simulink model "WL_test"  (R2025a)
settings: Solver=ode4  StartTime=0.0  StopTime=T_sim  FixedStep=Dt_sim  RelTol=1e-3
InitFcn:
  | % --- AVVIO AUTOMATICO PYTHON SERVER CON POP-UP (METODO FILE ROBUSTO) ---
  | fprintf('[Simulink] Preparazione simulazione...\n');
  | 
  | % 1. Pop-up per la Raffica
  | scelta_gust = questdlg('Vuoi includere la raffica (gust_H40.gust)?', ...
  |     'Configurazione Raffica', 'Si', 'No', 'No');
  | if isempty(scelta_gust), scelta_gust = 'No'; end
  | 
  | % 2. Pop-up per il Video
  | scelta_video = questdlg('Vuoi generare il video MP4 a fine simulazione?', ...
  |     'Configurazione Video', 'Si', 'No', 'No');
  | if isempty(scelta_video), scelta_video = 'No'; end
  | 
  | % --- PERCORSO ASSOLUTO ---
  | % Definiamo subito la cartella così MATLAB e WSL salvano e leggono dallo stesso posto
  | percorso = '/home/lpmatteo/Internship_INCARBONE_2026/LQR_first_controller_study/LQR_WL_simulation';
  | file_inputs = fullfile(percorso, 'python_inputs.txt');
  | 
  | % --- CREAZIONE FILE DI INPUT ---
  | fid = fopen(file_inputs, 'w');
  | fprintf(fid, '1\n'); % Scelta controller: 1 (LQI)
  | 
  | if strcmp(scelta_gust, 'Si')
  |     fprintf(fid, 's\n');
  | else
  |     fprintf(fid, 'n\n');
  | end
  | 
  | if strcmp(scelta_video, 'Si')
  |     % Se vogliamo il video, precompiliamo anche formato (mp4), qualità (high)
  |     % e la "Y" finale per far partire il render ASWING in automatico.
  |     fprintf(fid, 's\ngif\nmedium\nY\n');
  | else
  |     fprintf(fid, 'n\n');
  | end
  | fclose(fid);
  | 
  | % --- AVVIO DEL SERVER WSL ---
  | % Diciamo a Python di prendere le risposte direttamente dal file appena creato
  | cmd_wsl = sprintf('start "WingLoop Python Server" wsl -e bash -ic "cd %s && conda activate WINGLOOP && python3 controller_wingloop.py < python_inputs.txt; exec bash"', percorso);
  | 
  | system(cmd_wsl);
values from neighbouring files (symbols this model uses):
  E2ref = 23.6475887    [WL_main.m]
  F2ref = -6.63806152    [WL_main.m]
  t_int = 0.5    [WL_main.m]
  tau = 0.1    [WL_main.m]
  u_trim = [0, F2ref, F3ref, 0, E2ref, E2ref]    [WL_main.m]
undefined symbols (not defined in the file or in its folder): DiscIntNeverNeededParam, FullModel, idx, K_i, K_wu, K_z, matrices, ref_vec, ref_vecP, ROM, sat_engine
libraries: cstblocks x1
settings Model: SimulationMode=accelerator  Creator=lpmat  LastModifiedBy=lpmat

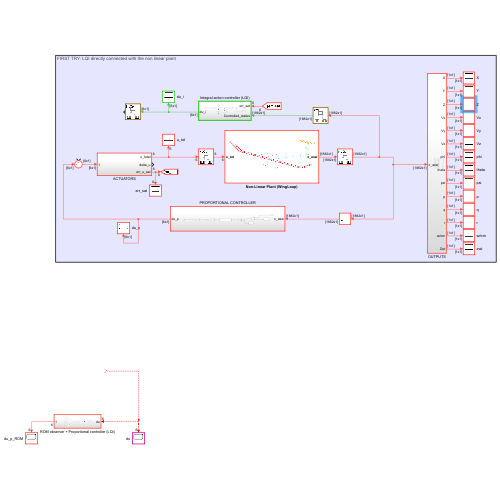
[thumbnail: Simulink's stored preview of the top-level diagram]
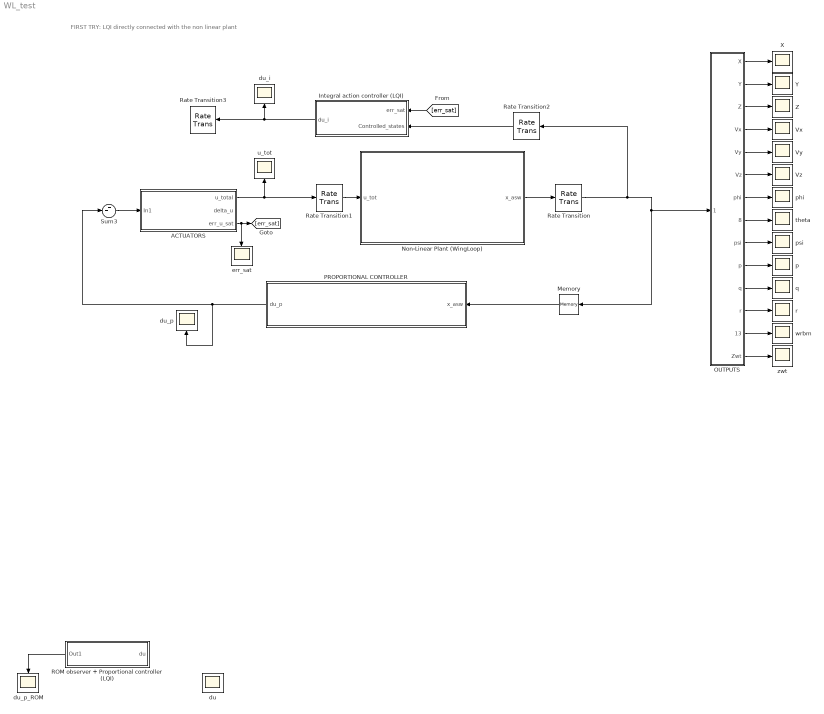
== system WL_test ==
  note: FIRST TRY: LQI directly connected with the non linear plant
  ACTUATORS : Subsystem
  Integral action controller (LQI) : Subsystem  TreatAsAtomicUnit=on  SystemSampleTime=t_int
  Memory : Memory  InitialCondition=FullModel.X0
  Non-Linear Plant (WingLoop) : Subsystem
      mask Display: image('Screenshot 2026-03-18 123158.png');
  OUTPUTS : Subsystem
  PROPORTIONAL CONTROLLER : Subsystem
  ROM observer + Proportional controller (LQI) : Subsystem
  Rate Transition : RateTransition  InitialCondition=FullModel.X0  OutPortSampleTime=Ts_control
  Rate Transition1 : RateTransition  InitialCondition=u_trim  OutPortSampleTime=Dt_asw
  Rate Transition2 : RateTransition  InitialCondition=FullModel.X0  OutPortSampleTime=t_int
  Rate Transition3 : RateTransition  OutPortSampleTime=Ts_control
  Sum3 : Sum  Inputs=--|
  Vx : Scope
      settings: ActiveDisplayYMinimum=-30.667463075  ActiveDisplayYMaximum=-29.643238325000002  DataLoggingVariableName=ScopeData9
  Vy : Scope
      settings: ActiveDisplayYMinimum=-0.022981843775  ActiveDisplayYMaximum=0.019016099975  DataLoggingVariableName=ScopeData2
  Vz : Scope
      settings: ActiveDisplayYMinimum=-4.1942458462499994  ActiveDisplayYMaximum=3.14147451625  DataLoggingVariableName=ScopeData23
  X : Scope
      settings: ActiveDisplayYMinimum=-3445.898072785  ActiveDisplayYMaximum=379.55975506499993
  Y : Scope
      settings: ActiveDisplayYMinimum=-11.715700294646378  ActiveDisplayYMaximum=7.8645535005168945
  Z : Scope
      settings: ActiveDisplayYMinimum=-2.916242765  ActiveDisplayYMaximum=10.900665085  DataLoggingVariableName=ScopeData11
  du : Scope
      settings: ActiveDisplayYMinimum=-1  ActiveDisplayYMaximum=1  DataLoggingVariableName=ScopeData15
  du_i : Scope
      settings: ActiveDisplayYMinimum=-0.0019582531234373637  ActiveDisplayYMaximum=0.0017838770388506043  DataLoggingVariableName=ScopeData5
  du_p : Scope
      settings: ActiveDisplayYMinimum=-2.2212573201433456  ActiveDisplayYMaximum=2.0941100207489196  DataLoggingVariableName=ScopeData13
  du_p_ROM : Scope
      settings: ActiveDisplayYMinimum=-1  ActiveDisplayYMaximum=1  DataLoggingVariableName=ScopeData10
  err_sat : Scope
      settings: ActiveDisplayYMinimum=-1  ActiveDisplayYMaximum=1  DataLoggingVariableName=ScopeData6
  p : Scope
      settings: ActiveDisplayYMinimum=-0.0001631406245  ActiveDisplayYMaximum=0.0001678073805  DataLoggingVariableName=ScopeData7
  phi : Scope
      settings: ActiveDisplayYMinimum=-4.954931666598749E-6  ActiveDisplayYMaximum=4.4625239296288751E-5  DataLoggingVariableName=ScopeData3
  psi : Scope
      settings: ActiveDisplayYMinimum=-2.941824858275E-5  ActiveDisplayYMaximum=3.8845402447499991E-6  DataLoggingVariableName=ScopeData4
  q : Scope
      settings: ActiveDisplayYMinimum=-0.1020126258875  ActiveDisplayYMaximum=0.12159143298749998  DataLoggingVariableName=ScopeData25
  r : Scope
      settings: ActiveDisplayYMinimum=-9.1499201112499989E-7  ActiveDisplayYMaximum=3.502066890125E-6  DataLoggingVariableName=ScopeData8
  theta : Scope
      settings: ActiveDisplayYMinimum=-0.557096708875  ActiveDisplayYMaximum=0.62679834987499994  DataLoggingVariableName=ScopeData14
  u_tot : Scope
      settings: ActiveDisplayYMinimum=-15.360293933915493  ActiveDisplayYMaximum=27.981801998175822  DataLoggingVariableName=ScopeData12
  wrbm : Scope
      settings: ActiveDisplayYMinimum=4.1562448775  ActiveDisplayYMaximum=36.6690849025  DataLoggingVariableName=ScopeData26
  zwt : Scope
      settings: ActiveDisplayYMinimum=2.5963466775  ActiveDisplayYMaximum=6.8764531025  DataLoggingVariableName=ScopeData16
  wires:
  Integral action controller (LQI)/1(du_i) -> Rate Transition3/1, du_i/1
  OUTPUTS/3(Z) -> Z/1
  OUTPUTS/4(Vx) -> Vx/1
  ACTUATORS/1(u_total) -> Rate Transition1/1, u_tot/1
  [err_sat] -> Integral action controller (LQI)/1(err_sat)
  Non-Linear Plant (WingLoop)/1(x_asw) -> Rate Transition/1
  OUTPUTS/8(theta) -> theta/1
  OUTPUTS/6(Vz) -> Vz/1
  OUTPUTS/11(q) -> q/1
  OUTPUTS/13(wrbm) -> wrbm/1
  OUTPUTS/1(X) -> X/1
  OUTPUTS/2(Y) -> Y/1
  OUTPUTS/5(Vy) -> Vy/1
  OUTPUTS/7(phi) -> phi/1
  OUTPUTS/9(psi) -> psi/1
  OUTPUTS/10(p) -> p/1
  OUTPUTS/12(r) -> r/1
  ACTUATORS/3(err_u_sat) -> err_sat/1, [err_sat]
  Rate Transition/1 -> Memory/1, OUTPUTS/1(x_asw), Rate Transition2/1
  Rate Transition1/1 -> Non-Linear Plant (WingLoop)/1(u_tot)
  ROM observer + Proportional controller (LQI)/1(Out1) -> du_p_ROM/1
  ? -> ROM observer + Proportional controller (LQI)/1(du), du/1
  PROPORTIONAL CONTROLLER/1(du_p) -> Sum3/2, du_p/1
  OUTPUTS/14(Zwt) -> zwt/1
  Rate Transition2/1 -> Integral action controller (LQI)/2(Controlled_states)
  Memory/1 -> PROPORTIONAL CONTROLLER/1(x_asw)
  Sum3/1 -> ACTUATORS/1(In1)

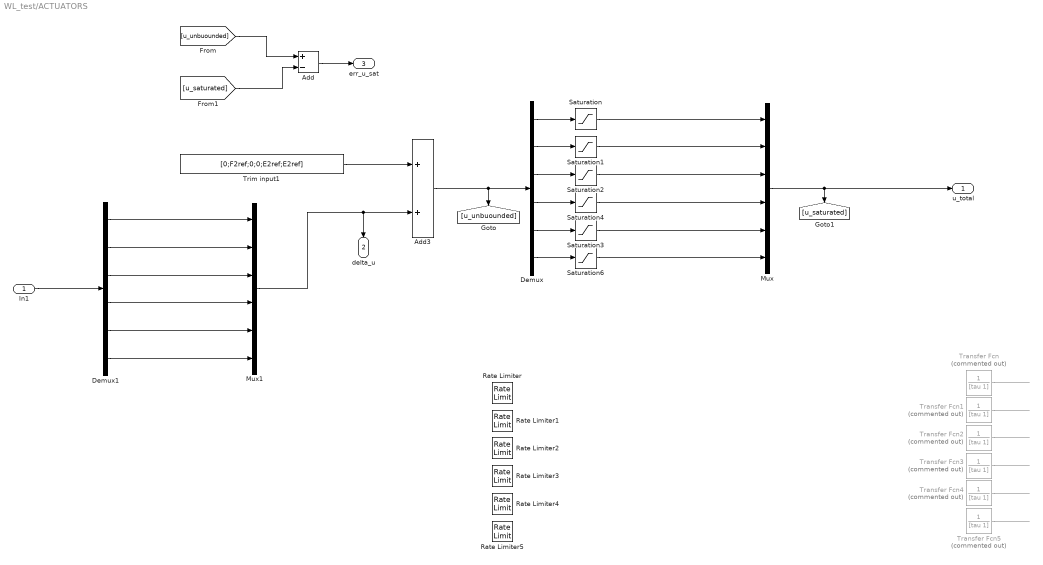
== system WL_test/ACTUATORS ==
  In1 : Inport
  Add : Sum  Inputs=+-
  Add3 : Sum
  Demux : Demux  Outputs=6
  Demux1 : Demux  Outputs=6
  Mux : Mux  Inputs=6
  Mux1 : Mux  Inputs=6
  Rate Limiter : RateLimiter  RisingSlewLimit=15  FallingSlewLimit=-15  SampleTimeMode=inherited  InitialCondition=u_trim(1)
  Rate Limiter1 : RateLimiter  RisingSlewLimit=15  FallingSlewLimit=-15  SampleTimeMode=inherited  InitialCondition=u_trim(2)
  Rate Limiter2 : RateLimiter  RisingSlewLimit=15  FallingSlewLimit=-15  SampleTimeMode=inherited  InitialCondition=u_trim(3)
  Rate Limiter3 : RateLimiter  RisingSlewLimit=15  FallingSlewLimit=-15  SampleTimeMode=inherited  InitialCondition=u_trim(4)
  Rate Limiter4 : RateLimiter  RisingSlewLimit=15  FallingSlewLimit=-15  SampleTimeMode=inherited  InitialCondition=u_trim(5)
  Rate Limiter5 : RateLimiter  RisingSlewLimit=15  FallingSlewLimit=-15  SampleTimeMode=inherited  InitialCondition=u_trim(6)
  Saturation{,1..2,4} (4 alike) : Saturate  UpperLimit=15  LowerLimit=-15
  Saturation3 : Saturate  UpperLimit=abs(E2ref)+abs(sat_engine)  LowerLimit=-(abs(E2ref)+abs(sat_engine))
  Saturation6 : Saturate  UpperLimit=abs(E2ref)+abs(sat_engine)  LowerLimit=-(abs(E2ref)+abs(sat_engine))
  Transfer Fcn{,1..5} (6 alike) : TransferFcn  Commented=on  Denominator=[tau 1]
  Trim input1 : Constant  Value=[0;F2ref;0;0;E2ref;E2ref]
  u_total : Outport
  delta_u : Outport  Port=2
  err_u_sat : Outport  Port=3
  wires:
  Trim input1/1 -> Add3/1
  Add3/1 -> Demux/1, [u_unbuounded]
  Demux/1 -> Saturation/1
  Demux/2 -> Saturation1/1
  Demux/3 -> Saturation2/1
  Demux/4 -> Saturation4/1
  Demux/5 -> Saturation3/1
  Demux/6 -> Saturation6/1
  Mux/1 -> u_total/1, [u_saturated]
  [u_unbuounded] -> Add/1
  [u_saturated] -> Add/2
  Add/1 -> err_u_sat/1
  In1/1 -> Demux1/1
  Demux1/1 -> Mux1/1
  Demux1/2 -> Mux1/2
  Demux1/3 -> Mux1/3
  Demux1/4 -> Mux1/4
  Demux1/5 -> Mux1/5
  Demux1/6 -> Mux1/6
  Mux1/1 -> Add3/2, delta_u/1
  Transfer Fcn1/1 -> ?
  ? -> Transfer Fcn3/1
  Transfer Fcn3/1 -> ?
  ? -> Transfer Fcn1/1
  ? -> Transfer Fcn2/1
  ? -> Transfer Fcn4/1
  Transfer Fcn4/1 -> ?
  ? -> Transfer Fcn/1
  Transfer Fcn/1 -> ?
  Transfer Fcn2/1 -> ?
  Transfer Fcn5/1 -> ?
  ? -> Transfer Fcn5/1
  Saturation6/1 -> Mux/6
  Saturation3/1 -> Mux/5
  Saturation4/1 -> Mux/4
  Saturation2/1 -> Mux/3
  Saturation1/1 -> Mux/2
  Saturation/1 -> Mux/1

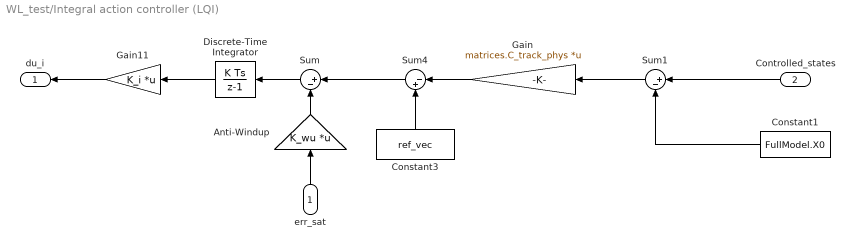
== system WL_test/Integral action controller (LQI) ==
  err_sat : Inport
  Controlled_states : Inport  Port=2
  Anti-Windup : Gain  Gain=K_wu  Multiplication=Matrix(K*u)
  Constant1 : Constant  Value=FullModel.X0
  Constant3 : Constant  Value=ref_vec
  Discrete-Time Integrator : DiscreteIntegrator  SampleTime=-1  LimitOutput=on  UpperSaturationLimit=10  LowerSaturationLimit=-10  ICPrevOutput=DiscIntNeverNeededParam  ICPrevScaledInput=DiscIntNeverNeededParam
  Gain : Gain  Gain=matrices.C_track_phys  Multiplication=Matrix(K*u)
  Gain11 : Gain  Gain=K_i  Multiplication=Matrix(K*u)
  Sum : Sum  Inputs=|+-
  Sum1 : Sum  Inputs=|+-
  Sum4 : Sum  Inputs=|-+
  du_i : Outport
  wires:
  Gain11/1 -> du_i/1
  Gain/1 -> Sum4/1
  Sum1/1 -> Gain/1
  Discrete-Time Integrator/1 -> Gain11/1
  Constant3/1 -> Sum4/2
  Sum4/1 -> Sum/1
  err_sat/1 -> Anti-Windup/1
  Sum/1 -> Discrete-Time Integrator/1
  Anti-Windup/1 -> Sum/2
  Constant1/1 -> Sum1/2
  Controlled_states/1 -> Sum1/1

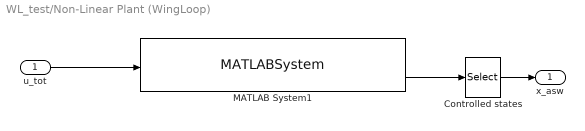
== system WL_test/Non-Linear Plant (WingLoop) ==
  u_tot : Inport
  Controlled states : Selector  InputPortWidth=1888  IndexOptions=Index vector (dialog)  Indices=[1:1882]  OutputSizes=1
  MATLAB System1 : MATLABSystem  System=AswingPlant  ServerHost=localhost  ServerPort=5005  NumModalStates=ROM.n_modal  NumPhysicalStates=FullModel.n_orig+ FullModel.n_in  SimulateUsing=Interpreted execution
      mask Type: AswingPlant
  x_asw : Outport
  wires:
  MATLAB System1/2 -> Controlled states/1
  u_tot/1 -> MATLAB System1/1
  Controlled states/1 -> x_asw/1

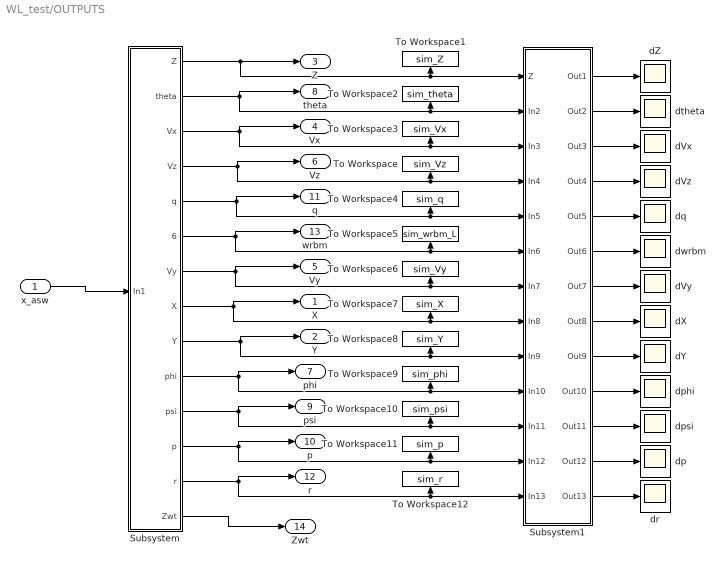
== system WL_test/OUTPUTS ==
  x_asw : Inport
  Subsystem : Subsystem
  Subsystem1 : Subsystem
  To Workspace : ToWorkspace  VariableName=sim_Vz  SaveFormat=Timeseries  SampleTime=-1
  To Workspace1 : ToWorkspace  VariableName=sim_Z  SaveFormat=Timeseries  SampleTime=-1
  To Workspace10 : ToWorkspace  VariableName=sim_psi  SaveFormat=Timeseries  SampleTime=-1
  To Workspace11 : ToWorkspace  VariableName=sim_p  SaveFormat=Timeseries  SampleTime=-1
  To Workspace12 : ToWorkspace  VariableName=sim_r  SaveFormat=Timeseries  SampleTime=-1
  To Workspace2 : ToWorkspace  VariableName=sim_theta  SaveFormat=Timeseries  SampleTime=-1
  To Workspace3 : ToWorkspace  VariableName=sim_Vx  SaveFormat=Timeseries  SampleTime=-1
  To Workspace4 : ToWorkspace  VariableName=sim_q  SaveFormat=Timeseries  SampleTime=-1
  To Workspace5 : ToWorkspace  VariableName=sim_wrbm_L  SaveFormat=Timeseries  SampleTime=-1
  To Workspace6 : ToWorkspace  VariableName=sim_Vy  SaveFormat=Timeseries  SampleTime=-1
  To Workspace7 : ToWorkspace  VariableName=sim_X  SaveFormat=Timeseries  SampleTime=-1
  To Workspace8 : ToWorkspace  VariableName=sim_Y  SaveFormat=Timeseries  SampleTime=-1
  To Workspace9 : ToWorkspace  VariableName=sim_phi  SaveFormat=Timeseries  SampleTime=-1
  dVx : Scope
      settings: ActiveDisplayYMinimum=29.833222698725  ActiveDisplayYMaximum=29.833684327474998  DataLoggingVariableName=ScopeData17
  dVy : Scope
      settings: ActiveDisplayYMinimum=-0.014985325000000046  ActiveDisplayYMaximum=0.13486792500000044  DataLoggingVariableName=ScopeData35
  dVz : Scope
      settings: ActiveDisplayYMinimum=-0.014985325000000046  ActiveDisplayYMaximum=0.13486792500000044  DataLoggingVariableName=ScopeData22
  dX : Scope
      settings: ActiveDisplayYMinimum=-0.014985325000000046  ActiveDisplayYMaximum=0.13486792500000044  DataLoggingVariableName=ScopeData35
  dY : Scope
      settings: ActiveDisplayYMinimum=-0.014985325000000046  ActiveDisplayYMaximum=0.13486792500000044  DataLoggingVariableName=ScopeData17
  dZ : Scope
      settings: ActiveDisplayYMinimum=-1  ActiveDisplayYMaximum=1  DataLoggingVariableName=ScopeData21
  dp : Scope
      settings: ActiveDisplayYMinimum=-0.014985325000000046  ActiveDisplayYMaximum=0.13486792500000044  DataLoggingVariableName=ScopeData21
  dphi : Scope
      settings: ActiveDisplayYMinimum=-0.014985325000000046  ActiveDisplayYMaximum=0.13486792500000044  DataLoggingVariableName=ScopeData17
  dpsi : Scope
      settings: ActiveDisplayYMinimum=-0.014985325000000046  ActiveDisplayYMaximum=0.13486792500000044  DataLoggingVariableName=ScopeData20
  dq : Scope
      settings: ActiveDisplayYMinimum=-0.014985325000000046  ActiveDisplayYMaximum=0.13486792500000044  DataLoggingVariableName=ScopeData24
  dr : Scope
      settings: ActiveDisplayYMinimum=-0.014985325000000046  ActiveDisplayYMaximum=0.13486792500000044  DataLoggingVariableName=ScopeData21
  dtheta : Scope
      settings: ActiveDisplayYMinimum=-0.338013509575  ActiveDisplayYMaximum=0.091025734174999984  DataLoggingVariableName=ScopeData20
  dwrbm : Scope
      settings: ActiveDisplayYMinimum=-0.014985325000000046  ActiveDisplayYMaximum=0.13486792500000044  DataLoggingVariableName=ScopeData27
  X : Outport
  Y : Outport  Port=2
  Z : Outport  Port=3
  Vx : Outport  Port=4
  Vy : Outport  Port=5
  Vz : Outport  Port=6
  phi : Outport  Port=7
  theta : Outport  Port=8
  psi : Outport  Port=9
  p : Outport  Port=10
  q : Outport  Port=11
  r : Outport  Port=12
  wrbm : Outport  Port=13
  Zwt : Outport  Port=14
  wires:
  Subsystem/5(q) -> Subsystem1/5(In5), To Workspace4/1, q/1
  Subsystem/2(theta) -> To Workspace2/1, Subsystem1/2(In2), theta/1
  Subsystem/4(Vz) -> Subsystem1/4(In4), To Workspace/1, Vz/1
  Subsystem/6(wrbm_L) -> Subsystem1/6(In6), To Workspace5/1, wrbm/1
  Subsystem/3(Vx) -> To Workspace3/1, Subsystem1/3(In3), Vx/1
  Subsystem/7(Vy) -> To Workspace6/1, Subsystem1/7(In7), Vy/1
  Subsystem/11(psi) -> Subsystem1/11(In11), To Workspace10/1, psi/1
  Subsystem/13(r) -> Subsystem1/13(In13), To Workspace12/1, r/1
  Subsystem/9(Y) -> Subsystem1/9(In9), To Workspace8/1, Y/1
  Subsystem/12(p) -> To Workspace11/1, Subsystem1/12(In12), p/1
  Subsystem/8(X) -> To Workspace7/1, Subsystem1/8(In8), X/1
  Subsystem/10(phi) -> To Workspace9/1, Subsystem1/10(In10), phi/1
  x_asw/1 -> Subsystem/1(In1)
  Subsystem/1(Z) -> To Workspace1/1, Subsystem1/1(Z), Z/1
  Subsystem1/1(Out1) -> dZ/1
  Subsystem1/2(Out2) -> dtheta/1
  Subsystem1/3(Out3) -> dVx/1
  Subsystem1/4(Out4) -> dVz/1
  Subsystem1/5(Out5) -> dq/1
  Subsystem1/6(Out6) -> dwrbm/1
  Subsystem1/7(Out7) -> dVy/1
  Subsystem1/8(Out8) -> dX/1
  Subsystem1/9(Out9) -> dY/1
  Subsystem1/10(Out10) -> dphi/1
  Subsystem1/11(Out11) -> dpsi/1
  Subsystem1/12(Out12) -> dp/1
  Subsystem1/13(Out13) -> dr/1
  Subsystem/14(Zwt) -> Zwt/1

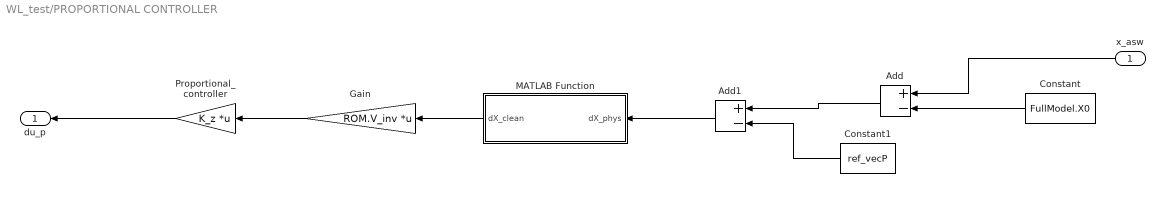
== system WL_test/PROPORTIONAL CONTROLLER ==
  x_asw : Inport
  Add : Sum  Inputs=+-
  Add1 : Sum  Inputs=+-
  Constant : Constant  Value=FullModel.X0
  Constant1 : Constant  Value=ref_vecP
  Gain : Gain  Gain=ROM.V_inv  Multiplication=Matrix(K*u)
  MATLAB Function : MATLAB Function  TreatAsAtomicUnit=on
  Proportional_controller : Gain  Gain=K_z  Multiplication=Matrix(K*u)
  du_p : Outport
  wires:
  x_asw/1 -> Add/1
  Gain/1 -> Proportional_controller/1
  Proportional_controller/1 -> du_p/1
  Constant/1 -> Add/2
  MATLAB Function/1(dX_clean) -> Gain/1
  Add1/1 -> MATLAB Function/1(dX_phys)
  Add/1 -> Add1/1
  Constant1/1 -> Add1/2

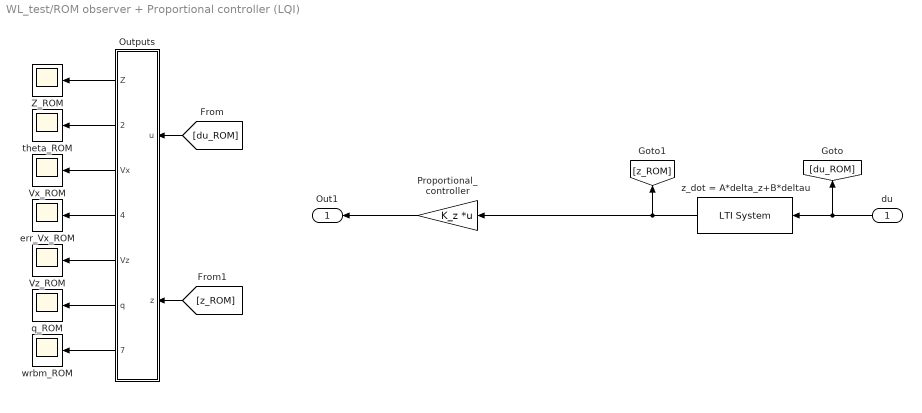
== system WL_test/ROM observer + Proportional controller (LQI) ==
  du : Inport
  Outputs : Subsystem
  Proportional_controller : Gain  Gain=K_z  Multiplication=Matrix(K*u)
  Vx_ROM : Scope
      settings: ActiveDisplayYMinimum=-29.75997799121388  ActiveDisplayYMaximum=-29.616858798151441  DataLoggingVariableName=ScopeData28
  Vz_ROM : Scope
      settings: ActiveDisplayYMinimum=-2.6148202510273633  ActiveDisplayYMaximum=-2.6136511943302931  DataLoggingVariableName=ScopeData29
  "Z_ROM " : Scope
      settings: ActiveDisplayYMinimum=-1.6253200350743973E-7  ActiveDisplayYMaximum=1.4627880315669578E-6  DataLoggingVariableName=ScopeData30
  err_Vx_ROM : Scope
      settings: ActiveDisplayYMinimum=-0.016507868182031336  ActiveDisplayYMaximum=0.11294531868689238  DataLoggingVariableName=ScopeData31
  q_ROM : Scope
      settings: ActiveDisplayYMinimum=-0.031623634831333659  ActiveDisplayYMaximum=0.0093452758439209  DataLoggingVariableName=ScopeData32
  theta_ROM : Scope
      settings: ActiveDisplayYMinimum=0.087579549883469346  ActiveDisplayYMaximum=0.088048251339121  DataLoggingVariableName=ScopeData33
  wrbm_ROM : Scope
      settings: ActiveDisplayYMinimum=17.5112693898615  ActiveDisplayYMaximum=17.875639730778097  DataLoggingVariableName=ScopeData34
  z_dot = A*delta_z+B*deltau : cstblocks/LTI System  sys=sys_fb  IC=0  PadeOrder=0
      link override Input Delay: Ts=-1
  Out1 : Outport
  wires:
  du/1 -> z_dot = A*delta_z+B*deltau/1, [du_ROM]
  Outputs/1(Z) -> "Z_ROM "/1
  Outputs/5(Vz) -> Vz_ROM/1
  Outputs/6(q) -> q_ROM/1
  Outputs/3(Vx) -> Vx_ROM/1
  Outputs/4(err_Vx) -> err_Vx_ROM/1
  Outputs/7(wrbm) -> wrbm_ROM/1
  Outputs/2(theta) -> theta_ROM/1
  [du_ROM] -> Outputs/1(u)
  [z_ROM] -> Outputs/2(z)
  Proportional_controller/1 -> Out1/1
  z_dot = A*delta_z+B*deltau/1 -> Proportional_controller/1, [z_ROM]

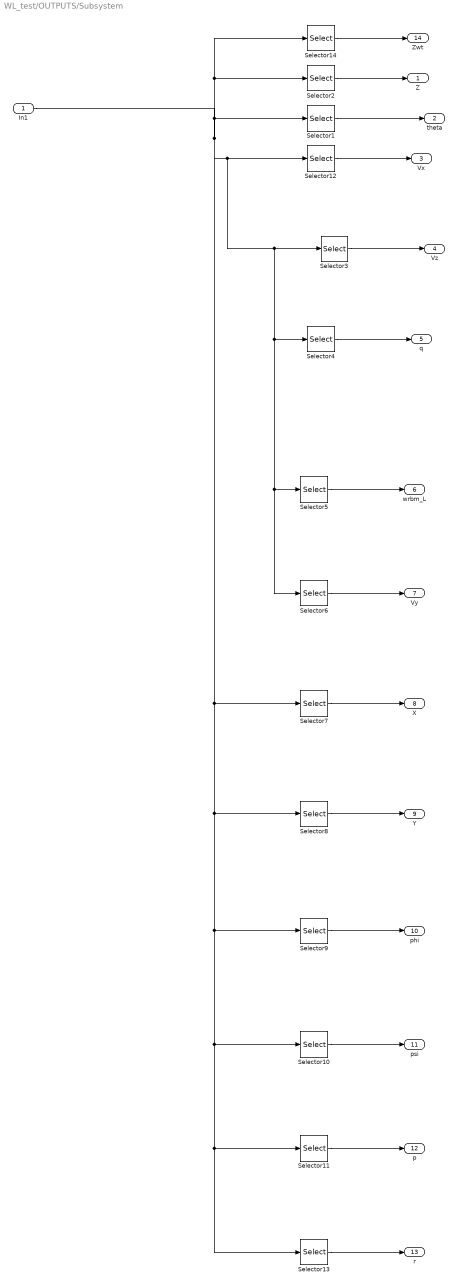
== system WL_test/OUTPUTS/Subsystem ==
  In1 : Inport
  Selector1 : Selector  InputPortWidth=1882  IndexOptions=Index vector (dialog)  Indices=[idx.theta]  OutputSizes=1
  Selector10 : Selector  InputPortWidth=1882  IndexOptions=Index vector (dialog)  Indices=[idx.psi]  OutputSizes=1
  Selector11 : Selector  InputPortWidth=1882  IndexOptions=Index vector (dialog)  Indices=[idx.p]  OutputSizes=1
  Selector12 : Selector  InputPortWidth=1882  IndexOptions=Index vector (dialog)  Indices=[idx.Vx]  OutputSizes=1
  Selector13 : Selector  InputPortWidth=1882  IndexOptions=Index vector (dialog)  Indices=[idx.r]  OutputSizes=1
  Selector14 : Selector  InputPortWidth=1882  IndexOptions=Index vector (dialog)  Indices=[idx.Zwt]  OutputSizes=1
  Selector2 : Selector  InputPortWidth=1882  IndexOptions=Index vector (dialog)  Indices=[idx.Z]  OutputSizes=1
  Selector3 : Selector  InputPortWidth=1882  IndexOptions=Index vector (dialog)  Indices=[idx.Vz]  OutputSizes=1
  Selector4 : Selector  InputPortWidth=1882  IndexOptions=Index vector (dialog)  Indices=[idx.q]  OutputSizes=1
  Selector5 : Selector  InputPortWidth=1882  IndexOptions=Index vector (dialog)  Indices=[idx.wrbm_L]  OutputSizes=1
  Selector6 : Selector  InputPortWidth=1882  IndexOptions=Index vector (dialog)  Indices=[idx.Vy]  OutputSizes=1
  Selector7 : Selector  InputPortWidth=1882  IndexOptions=Index vector (dialog)  Indices=[idx.X]  OutputSizes=1
  Selector8 : Selector  InputPortWidth=1882  IndexOptions=Index vector (dialog)  Indices=[idx.Y]  OutputSizes=1
  Selector9 : Selector  InputPortWidth=1882  IndexOptions=Index vector (dialog)  Indices=[idx.phi]  OutputSizes=1
  Z : Outport
  theta : Outport  Port=2
  Vx : Outport  Port=3
  Vz : Outport  Port=4
  q : Outport  Port=5
  wrbm_L : Outport  Port=6
  Vy : Outport  Port=7
  X : Outport  Port=8
  Y : Outport  Port=9
  phi : Outport  Port=10
  psi : Outport  Port=11
  p : Outport  Port=12
  r : Outport  Port=13
  Zwt : Outport  Port=14
  wires:
  Selector5/1 -> wrbm_L/1
  In1/1 -> Selector6/1, Selector5/1, Selector4/1, Selector3/1, Selector12/1, Selector14/1, Selector2/1, Selector1/1, Selector13/1, Selector11/1, Selector10/1, Selector9/1, Selector8/1, Selector7/1
  Selector2/1 -> Z/1
  Selector3/1 -> Vz/1
  Selector9/1 -> phi/1
  Selector6/1 -> Vy/1
  Selector12/1 -> Vx/1
  Selector4/1 -> q/1
  Selector1/1 -> theta/1
  Selector10/1 -> psi/1
  Selector13/1 -> r/1
  Selector8/1 -> Y/1
  Selector11/1 -> p/1
  Selector7/1 -> X/1
  Selector14/1 -> Zwt/1

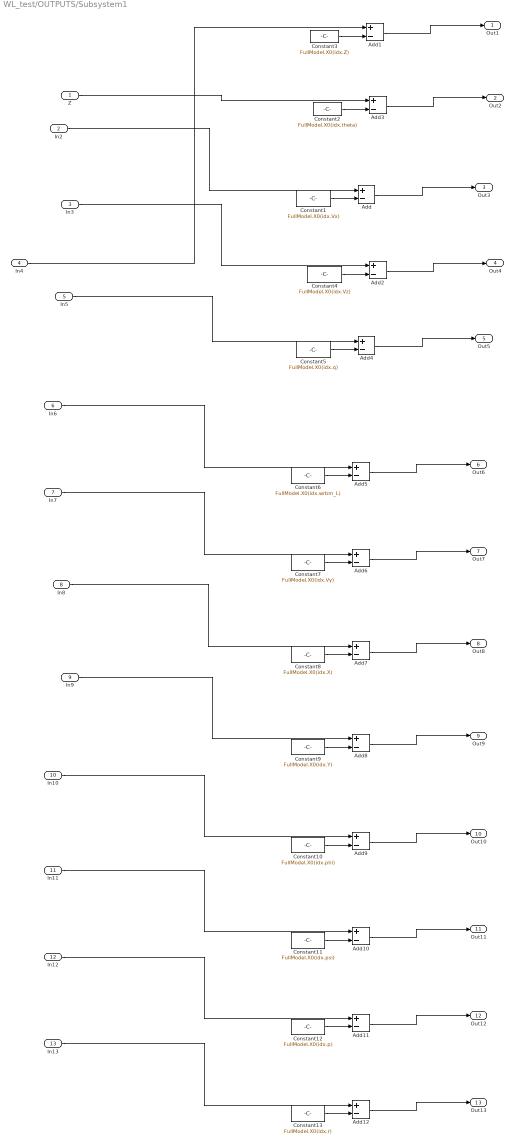
== system WL_test/OUTPUTS/Subsystem1 ==
  Z : Inport
  In2 : Inport  Port=2
  In3 : Inport  Port=3
  In4 : Inport  Port=4
  In5 : Inport  Port=5
  In6 : Inport  Port=6
  In7 : Inport  Port=7
  In8 : Inport  Port=8
  In9 : Inport  Port=9
  In10 : Inport  Port=10
  In11 : Inport  Port=11
  In12 : Inport  Port=12
  In13 : Inport  Port=13
  Add{,1..12} (13 alike) : Sum  Inputs=+-
  Constant1 : Constant  Value=FullModel.X0(idx.Vx)
  Constant10 : Constant  Value=FullModel.X0(idx.phi)
  Constant11 : Constant  Value=FullModel.X0(idx.psi)
  Constant12 : Constant  Value=FullModel.X0(idx.p)
  Constant13 : Constant  Value=FullModel.X0(idx.r)
  Constant2 : Constant  Value=FullModel.X0(idx.theta)
  Constant3 : Constant  Value=FullModel.X0(idx.Z)
  Constant4 : Constant  Value=FullModel.X0(idx.Vz)
  Constant5 : Constant  Value=FullModel.X0(idx.q)
  Constant6 : Constant  Value=FullModel.X0(idx.wrbm_L)
  Constant7 : Constant  Value=FullModel.X0(idx.Vy)
  Constant8 : Constant  Value=FullModel.X0(idx.X)
  Constant9 : Constant  Value=FullModel.X0(idx.Y)
  Out1 : Outport
  Out2 : Outport  Port=2
  Out3 : Outport  Port=3
  Out4 : Outport  Port=4
  Out5 : Outport  Port=5
  Out6 : Outport  Port=6
  Out7 : Outport  Port=7
  Out8 : Outport  Port=8
  Out9 : Outport  Port=9
  Out10 : Outport  Port=10
  Out11 : Outport  Port=11
  Out12 : Outport  Port=12
  Out13 : Outport  Port=13
  wires:
  Constant6/1 -> Add5/2
  Constant3/1 -> Add1/2
  In5/1 -> Add4/1
  In13/1 -> Add12/1
  Z/1 -> Add3/1
  Constant5/1 -> Add4/2
  Constant4/1 -> Add2/2
  Add5/1 -> Out6/1
  Constant1/1 -> Add/2
  In8/1 -> Add7/1
  In11/1 -> Add10/1
  Constant2/1 -> Add3/2
  Add12/1 -> Out13/1
  In3/1 -> Add2/1
  Add8/1 -> Out9/1
  Constant7/1 -> Add6/2
  In10/1 -> Add9/1
  Constant11/1 -> Add10/2
  Constant13/1 -> Add12/2
  Add4/1 -> Out5/1
  Add1/1 -> Out1/1
  Add7/1 -> Out8/1
  Constant9/1 -> Add8/2
  Constant12/1 -> Add11/2
  Constant8/1 -> Add7/2
  Add/1 -> Out3/1
  Constant10/1 -> Add9/2
  Add3/1 -> Out2/1
  In2/1 -> Add/1
  Add2/1 -> Out4/1
  Add11/1 -> Out12/1
  Add6/1 -> Out7/1
  Add10/1 -> Out11/1
  In12/1 -> Add11/1
  In4/1 -> Add1/1
  In7/1 -> Add6/1
  Add9/1 -> Out10/1
  In6/1 -> Add5/1
  In9/1 -> Add8/1

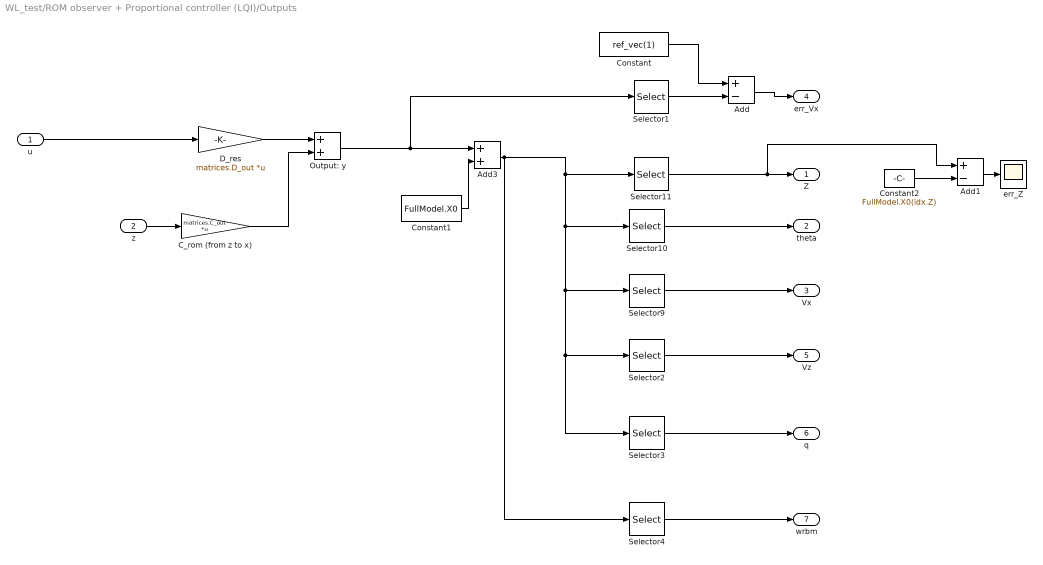
== system WL_test/ROM observer + Proportional controller (LQI)/Outputs ==
  u : Inport
  z : Inport  Port=2
  Add : Sum  Inputs=+-
  Add1 : Sum  Inputs=+-
  Add3 : Sum
  C_rom (from z to x) : Gain  Gain=matrices.C_out  Multiplication=Matrix(K*u)
  Constant : Constant  Value=ref_vec(1)
  Constant1 : Constant  Value=FullModel.X0
  Constant2 : Constant  Value=FullModel.X0(idx.Z)
  D_res : Gain  Gain=matrices.D_out  Multiplication=Matrix(K*u)
  Output: y : Sum
  Selector1 : Selector  InputPortWidth=1882  IndexOptions=Index vector (dialog)  Indices=[idx.Vx]  OutputSizes=1
  Selector10 : Selector  InputPortWidth=1882  IndexOptions=Index vector (dialog)  Indices=[idx.theta]  OutputSizes=1
  Selector11 : Selector  InputPortWidth=1882  IndexOptions=Index vector (dialog)  Indices=[idx.Z]  OutputSizes=1
  Selector2 : Selector  InputPortWidth=1882  IndexOptions=Index vector (dialog)  Indices=[idx.Vz]  OutputSizes=1
  Selector3 : Selector  InputPortWidth=1882  IndexOptions=Index vector (dialog)  Indices=[idx.q]  OutputSizes=1
  Selector4 : Selector  InputPortWidth=1882  IndexOptions=Index vector (dialog)  Indices=[idx.wrbm_L]  OutputSizes=1
  Selector9 : Selector  InputPortWidth=1882  IndexOptions=Index vector (dialog)  Indices=[idx.Vx]  OutputSizes=1
  err_Z : Scope
      settings: ActiveDisplayYMinimum=-0.52989229015549089  ActiveDisplayYMaximum=0.058876921128387862  DataLoggingVariableName=ScopeData20
  Z : Outport
  theta : Outport  Port=2
  Vx : Outport  Port=3
  err_Vx : Outport  Port=4
  Vz : Outport  Port=5
  q : Outport  Port=6
  wrbm : Outport  Port=7
  wires:
  C_rom (from z to x)/1 -> Output: y/2
  Constant1/1 -> Add3/2
  D_res/1 -> Output: y/1
  u/1 -> D_res/1
  Output: y/1 -> Selector1/1, Add3/1
  Selector10/1 -> theta/1
  z/1 -> C_rom (from z to x)/1
  Selector9/1 -> Vx/1
  Selector1/1 -> Add/2
  Add/1 -> err_Vx/1
  Constant/1 -> Add/1
  Selector11/1 -> Add1/1, Z/1
  Constant2/1 -> Add1/2
  Add1/1 -> err_Z/1
  Selector2/1 -> Vz/1
  Selector3/1 -> q/1
  Selector4/1 -> wrbm/1
  Add3/1 -> Selector4/1, Selector11/1, Selector10/1, Selector3/1, Selector2/1, Selector9/1

== matlab function WL_test/PROPORTIONAL CONTROLLER/MATLAB Function ==
  data: dX_phys input; dX_clean output
function dX_clean = mask_global_position(dX_phys)
    dX_clean = dX_phys;
    n_orig = 1882; 

    dX_clean(n_orig - 5) = 0; % Nasconde i Km percorsi in X
    
end
